simulink model "TST_DYN_AERO"  (Simulink 9.0)
settings: Solver=VariableStepAuto  StartTime=0.0  StopTime=10000  RelTol=1e-3
libraries: DYN_AERO x1, DYN_GRAV x1, DYN_TIME x1, DYN_TRA x1
settings Model: Creator=Mahal  LastModifiedBy=Mahal
settings DataIOCC: SaveFormat=Dataset
settings OptimizationCC: LifeSpan=auto
settings DebuggingCC: UnderspecifiedInitializationDetection=Simplified  MergeDetectMultiDrivingBlocksExec=error  SFUnexpectedBacktrackingDiag=error  SFNoUnconditionalDefaultTransitionDiag=error  SFExecutionAtInitializationDiag=warning
settings HardwareCC: ProdBitPerPointer=64  ProdBitPerSizeT=64  ProdBitPerPtrDiffT=64  ProdLargestAtomicFloat=Float  ProdIntDivRoundTo=Zero  ProdEndianess=LittleEndian  ProdWordSize=64  ProdHWDeviceType=Intel->x86-64 (Windows64)
settings ModelReferenceCC: PropagateSignalLabelsOutOfModel=on
settings CodeAppCC: StateflowObjectComments=off
settings GRTTargetCC: TargetLangStandard=C99 (ISO)
settings ConfigComp: CovMetricSettings=dwe  CovHtmlReporting=off  CovSaveCumulativeToWorkspaceVar=off  CovSaveSingleToWorkspaceVar=off  CovExternalEMLEnable=on

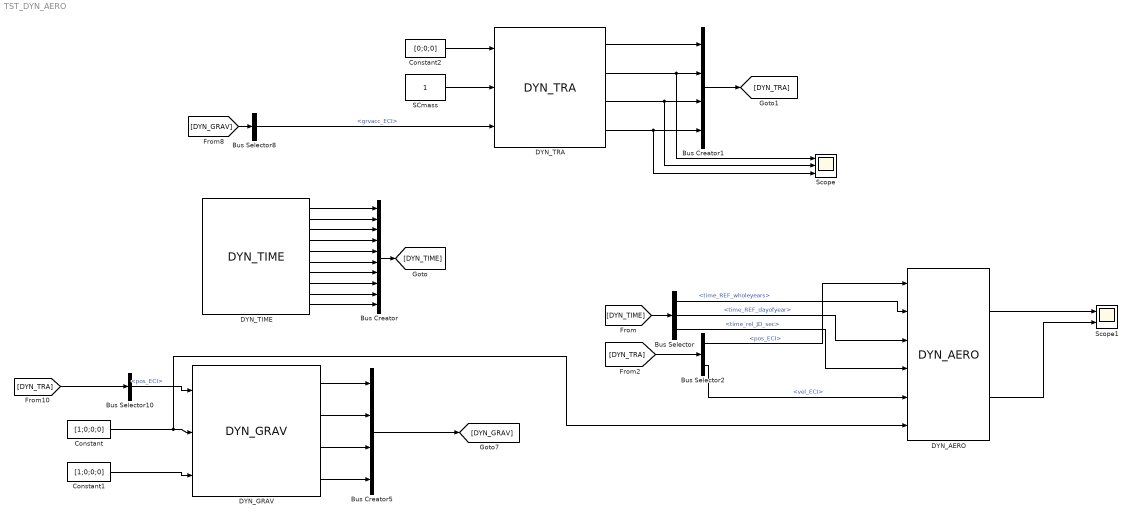
== system TST_DYN_AERO ==
  Bus Creator : BusCreator  Inputs=10
  Bus Creator1 : BusCreator  Inputs=4
  Bus Creator5 : BusCreator  Inputs=4
  Bus Selector : BusSelector  OutputSignals=time_REF_wholeyears,time_REF_dayofyear,time_rel_JD_sec
  Bus Selector10 : BusSelector  OutputSignals=pos_ECI
  Bus Selector2 : BusSelector  OutputSignals=pos_ECI,vel_ECI
  Bus Selector8 : BusSelector  OutputSignals=grvacc_ECI
  Constant : Constant  Value=[1;0;0;0]
  Constant1 : Constant  Value=[1;0;0;0]
  Constant2 : Constant  Value=[0;0;0]
  DYN_AERO : DYN_AERO/DYN_AERO
  DYN_GRAV : DYN_GRAV/DYN_GRAV
  DYN_TIME : DYN_TIME/DYN_TIME
  DYN_TRA : DYN_TRA/DYN_TRA
  SCmass : Constant
  Scope : Scope  NumInputPorts=3
  Scope1 : Scope  NumInputPorts=2
  wires:
  Bus Creator1/1 -> [DYN_TRA]
  DYN_TRA/4 -> Scope/3, Bus Creator1/4
  DYN_TRA/1 -> Bus Creator1/1
  DYN_TRA/2 -> Scope/1, Bus Creator1/2
  Constant2/1 -> DYN_TRA/1
  [DYN_GRAV] -> Bus Selector8/1
  SCmass/1 -> DYN_TRA/2
  DYN_TRA/3 -> Scope/2, Bus Creator1/3
  Bus Selector8/1 -> DYN_TRA/3  "<grvacc_ECI>"
  DYN_TIME/8 -> Bus Creator/8
  DYN_TIME/10 -> Bus Creator/10
  DYN_TIME/6 -> Bus Creator/6
  DYN_TIME/4 -> Bus Creator/4
  DYN_TIME/1 -> Bus Creator/1
  DYN_TIME/9 -> Bus Creator/9
  DYN_TIME/2 -> Bus Creator/2
  DYN_TIME/3 -> Bus Creator/3
  Bus Creator/1 -> [DYN_TIME]
  DYN_TIME/7 -> Bus Creator/7
  DYN_TIME/5 -> Bus Creator/5
  Bus Selector/3 -> DYN_AERO/4  "<time_rel_JD_sec>"
  Bus Selector/2 -> DYN_AERO/3  "<time_REF_dayofyear>"
  [DYN_TIME] -> Bus Selector/1
  [DYN_TRA] -> Bus Selector2/1
  Bus Selector/1 -> DYN_AERO/2  "<time_REF_wholeyears>"
  Bus Selector2/1 -> DYN_AERO/1  "<pos_ECI>"
  Bus Selector2/2 -> DYN_AERO/5  "<vel_ECI>"
  DYN_AERO/1 -> Scope1/1
  DYN_AERO/2 -> Scope1/2
  Constant/1 -> DYN_AERO/6, DYN_GRAV/2
  [DYN_TRA] -> Bus Selector10/1
  Constant1/1 -> DYN_GRAV/3
  Bus Creator5/1 -> [DYN_GRAV]
  DYN_GRAV/1 -> Bus Creator5/1
  DYN_GRAV/2 -> Bus Creator5/2
  DYN_GRAV/3 -> Bus Creator5/3
  Bus Selector10/1 -> DYN_GRAV/1  "<pos_ECI>"
  DYN_GRAV/4 -> Bus Creator5/4
